simulink model "c10_wp_snake"  (R2021b)
settings: Solver=FixedStepDiscrete  StartTime=0.0  StopTime=Inf  FixedStep=sampleTime  RelTol=1e-3  EnableMultiTasking=on
InitFcn:
  | sampleTime = 0.05;
  | nMedianSize=3;
  | % Robot parameters
  | % Robot parameters
  | wheelRadius = 0.0303;
  | robotRadius = 0.116*0.8;   %小车在仿真中显示的圆形的半径大小
  | Trackwidth = 0.0847;  %定义向量场直方图算法中小车的宽度
  | 
  | % Lidar parameters
  | sensorOffset = [0,0];
  | scanAngles = linspace(-pi/3,pi/3,20)';%y = linspace(x1,x2,n) 生成 n 个点。这些点的间距为 (x2-x1)/(n-1)。
  | maxRange = 0.2;
  | 
  | %%%%%%
  | ks=1;
  | 
  | init_pose_1=[0    0  0]';
  | init_pose_2=[0    0.2  -pi/2]';
  | init_pose_3=[0    0.4  -pi/2]';
  | init_pose_4=[0    0.6  -pi/2]';
  | init_pose_5=[0    0.8  -pi/2]';
  | init_pose_6=[0    1  -pi/2]';
  | init_pose_7=[0    1.2  -pi/2]';
  | init_pose_8=[0    1.4  -pi/2]';
  | init_pose_9=[0    1.6  -pi/2]';
  | init_pose_10=[0   1.8  -pi/2]';
  | 
  | % paremeters of pure persuit
  | desired_v=0.2;
  | desired_w=2*pi;
  | desired_lookahead=0.2;
  | kv=0;
  | kw=1;%加速转弯
  | GoalRadius=0.15;%到达目标判定阈值
  | 
  | % paremeters of recovery
  | %recovery_w=0.5
  | recovery_w=2;
  | % Vector Field Histogram
  | numSector=180;%Number of angular sector
  | vehicleRadius=robotRadius;
  | rangeDis=[ 0, 0 ];%Range distance limits (m):
  | thresholds=[ 3, 8 ];%Histogram thresholds
  | %binary histogram 大于8是障碍物，小于3是空白区
  | %Thresholds for computing binary histogram, specified as a two-element vector of scalars. The algorithm uses these thresholds to compute the binary histogram from the polar obstacle density. Polar obstacle density values higher than the upper threshold are represented as occupied space (1) in the binary histogram. Values smaller than the lower threshold are represented as free space (0). Values that fall between the limits are set to the values of a previous computed binary histogram if one exists from previous iterations. If a previous histogram does not exist, the value is set as free space (0).
  | safetyDis=0.1;%Safety distance
  | minimumTurningRadius=0.5*robotRadius;%Minimum turning radius (m):
undefined symbols (not defined in the file): Angular, DiscIntNeverNeededParam, Linear
libraries: robotlib x42, dspstat3 x30, robotalgslib x20
(part 1 of 5)
settings Model: Creator=The MathWorks, Inc.  LastModifiedBy=FCS
settings SolverCC: AlgebraicLoopSolver=TrustRegion
settings DataIOCC: LimitDataPoints=on  SaveFormat=Array  ReturnWorkspaceOutputs=off
settings OptimizationCC: EnhancedBackFolding=on  PassReuseOutputArgsAs=Individual arguments  ZeroExternalMemoryAtStartup=off  ZeroInternalMemoryAtStartup=off  MaxStackSize=64  OptimizeBlockOrder=speed  DifferentSizesBufferReuse=on  OptimizationCustomize=off  EfficientTunableParamExpr=on
settings DebuggingCC: SolverPrmCheckMsg=warning  ParameterTunabilityLossMsg=error  SFUnexpectedBacktrackingDiag=warning  SFNoUnconditionalDefaultTransitionDiag=warning  SFExecutionAtInitializationDiag=none  SFMachineParentedDataDiag=warning  ArithmeticOperatorsInVariantConditions=warning
settings HardwareCC: ProdBitPerPointer=32  ProdBitPerSizeT=32  ProdBitPerPtrDiffT=32  ProdLargestAtomicFloat=None  ProdIntDivRoundTo=Undefined  ProdEndianess=Unspecified  ProdWordSize=32  ProdHWDeviceType=Generic->Unspecified (assume 32-bit Generic)  TargetHWDeviceType=Generic->Unspecified (assume 32-bit Generic)
settings ModelReferenceCC: PropagateSignalLabelsOutOfModel=off
settings SFSimCC: SimUseLocalCustomCode=off  MATLABDynamicMemAllocThreshold=655360  CustomCodeUndefinedFunction=UseInterfaceOnly  SimTargetLang=C++
settings RTWCC: Description=Embedded Coder  SystemTargetFile=ert.tlc  HardwareBoard=Robot Operating System (ROS)  TLCOptions="-aInlineSetEventsForThisBaseRateFcn=TLC_FALSE -aSuppressMultiTaskScheduler=TLC_FALSE  -aRateBasedStepFcn=0"  TemplateMakefile=ert_default_tmf  RTWUseLocalCustomCode=off  Toolchain=Catkin  TargetLang=C++
settings CodeAppCC: ForceParamTrailComments=on  IgnoreCustomStorageClasses=off  OperatorAnnotations=on  SimulinkDataObjDesc=on  SFDataObjDesc=on  InsertBlockDesc=on
settings ERTTargetCC: SupportVariableSizeSignals=on
settings ConfigComp: CovMetricSettings=dw  CovSaveCumulativeToWorkspaceVar=on  CovSaveSingleToWorkspaceVar=on  CovExternalEMLEnable=off  CovSFcnEnable=off

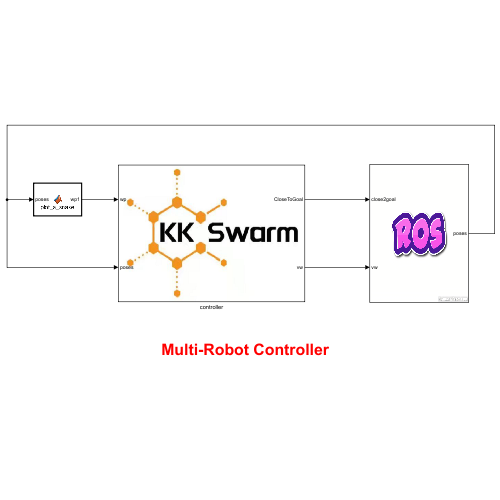
[thumbnail: Simulink's stored preview of the top-level diagram]
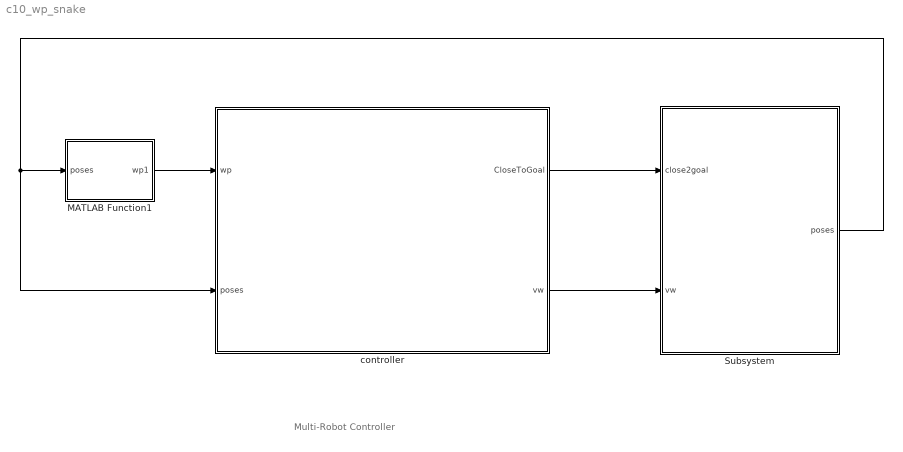
== system c10_wp_snake ==
  note: Multi-Robot Controller
  MATLAB Function1 : MATLAB Function  TreatAsAtomicUnit=on
  Subsystem : Subsystem
      mask Display: image('$imagefile'); % 使用工具条上的 "编辑图像" 进行更改。
  controller : Subsystem
      mask Display: image('$imagefile'); % 使用工具条上的 "编辑图像" 进行更改。
  wires:
  MATLAB Function1/1(wp1) -> controller/1(wp)
  controller/2(vw) -> Subsystem/2(vw)
  controller/1(CloseToGoal) -> Subsystem/1(close2goal)
  Subsystem/1(poses) -> controller/2(poses), MATLAB Function1/1(poses)

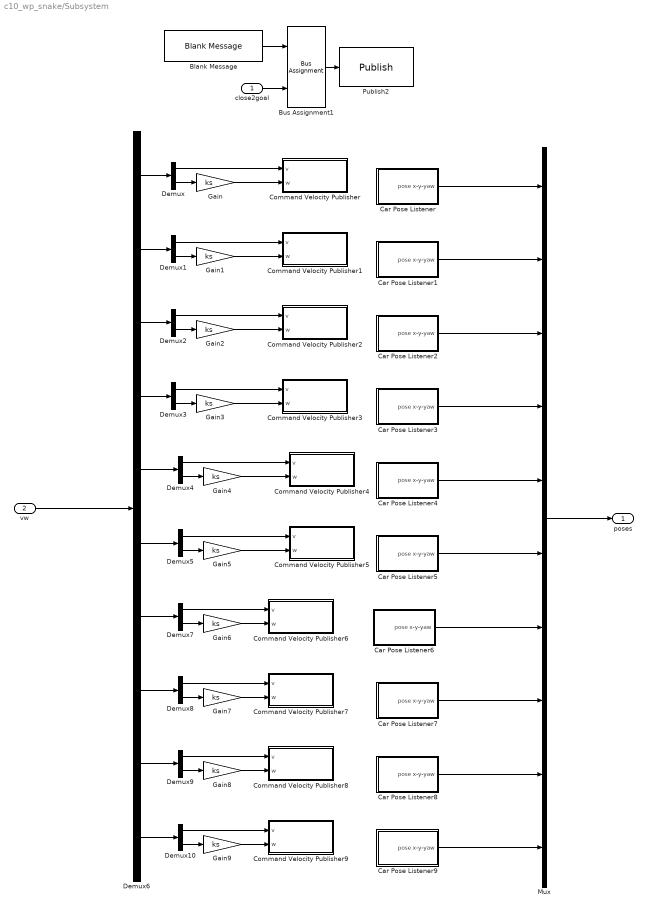
== system c10_wp_snake/Subsystem ==
  close2goal : Inport
  vw : Inport  Port=2
  Blank Message : robotlib/Blank Message  messageClass=Message  entityType=std_msgs/Float64  messageType=std_msgs/Float64  SampleTime=inf  legacyBusStruct=off
  Bus Assignment1 : BusAssignment  DialogController=Simulink.DDGSource_BusAssignment  AssignedSignals=Data
  Car Pose Listener : Subsystem
  Car Pose Listener1 : Subsystem
  Car Pose Listener2 : Subsystem
  Car Pose Listener3 : Subsystem
  Car Pose Listener4 : Subsystem
  Car Pose Listener5 : Subsystem
  Car Pose Listener6 : Subsystem
  Car Pose Listener7 : Subsystem
  Car Pose Listener8 : Subsystem
  Car Pose Listener9 : Subsystem
  Command Velocity Publisher : Subsystem
  Command Velocity Publisher1 : Subsystem
  Command Velocity Publisher2 : Subsystem
  Command Velocity Publisher3 : Subsystem
  Command Velocity Publisher4 : Subsystem
  Command Velocity Publisher5 : Subsystem
  Command Velocity Publisher6 : Subsystem
  Command Velocity Publisher7 : Subsystem
  Command Velocity Publisher8 : Subsystem
  Command Velocity Publisher9 : Subsystem
  Demux{,1..5,7..10} (10 alike) : Demux  Outputs=2
  Demux6 : Demux  Outputs=10
  Gain{,1..9} (10 alike) : Gain  Gain=ks
  Mux : Mux  Inputs=10
  Publish2 : robotlib/Publish  topicSource=Specify your own  topic=/close_goal  messageType=std_msgs/Float64  legacyBusStruct=off  messageQueueLength=105
  poses : Outport
  wires:
  Gain/1 -> Command Velocity Publisher/2(w)
  Demux/2 -> Gain/1
  Car Pose Listener/1(pose x-y-yaw) -> Mux/1
  Demux/1 -> Command Velocity Publisher/1(v)
  Car Pose Listener1/1(pose x-y-yaw) -> Mux/2
  Gain1/1 -> Command Velocity Publisher1/2(w)
  Demux1/2 -> Gain1/1
  Demux1/1 -> Command Velocity Publisher1/1(v)
  Car Pose Listener2/1(pose x-y-yaw) -> Mux/3
  Gain2/1 -> Command Velocity Publisher2/2(w)
  Demux2/2 -> Gain2/1
  Demux2/1 -> Command Velocity Publisher2/1(v)
  Car Pose Listener3/1(pose x-y-yaw) -> Mux/4
  Gain3/1 -> Command Velocity Publisher3/2(w)
  Demux3/2 -> Gain3/1
  Demux3/1 -> Command Velocity Publisher3/1(v)
  Gain4/1 -> Command Velocity Publisher4/2(w)
  Demux6/5 -> Demux4/1
  Demux4/2 -> Gain4/1
  Demux4/1 -> Command Velocity Publisher4/1(v)
  Car Pose Listener5/1(pose x-y-yaw) -> Mux/6
  Gain5/1 -> Command Velocity Publisher5/2(w)
  Demux6/6 -> Demux5/1
  Demux5/2 -> Gain5/1
  Demux5/1 -> Command Velocity Publisher5/1(v)
  Bus Assignment1/1 -> Publish2/1
  Blank Message/1 -> Bus Assignment1/1
  close2goal/1 -> Bus Assignment1/2
  Demux6/1 -> Demux/1
  Demux6/2 -> Demux1/1
  Demux6/3 -> Demux2/1
  Demux6/4 -> Demux3/1
  Car Pose Listener6/1(pose x-y-yaw) -> Mux/7
  Demux7/1 -> Command Velocity Publisher6/1(v)
  Demux7/2 -> Gain6/1
  Gain6/1 -> Command Velocity Publisher6/2(w)
  Demux6/7 -> Demux7/1
  Car Pose Listener7/1(pose x-y-yaw) -> Mux/8
  Demux8/1 -> Command Velocity Publisher7/1(v)
  Demux8/2 -> Gain7/1
  Gain7/1 -> Command Velocity Publisher7/2(w)
  Demux6/8 -> Demux8/1
  Car Pose Listener8/1(pose x-y-yaw) -> Mux/9
  Demux9/1 -> Command Velocity Publisher8/1(v)
  Demux9/2 -> Gain8/1
  Gain8/1 -> Command Velocity Publisher8/2(w)
  Demux6/9 -> Demux9/1
  Car Pose Listener9/1(pose x-y-yaw) -> Mux/10
  Demux10/1 -> Command Velocity Publisher9/1(v)
  Demux10/2 -> Gain9/1
  Gain9/1 -> Command Velocity Publisher9/2(w)
  Demux6/10 -> Demux10/1
  vw/1 -> Demux6/1
  Car Pose Listener4/1(pose x-y-yaw) -> Mux/5
  Mux/1 -> poses/1

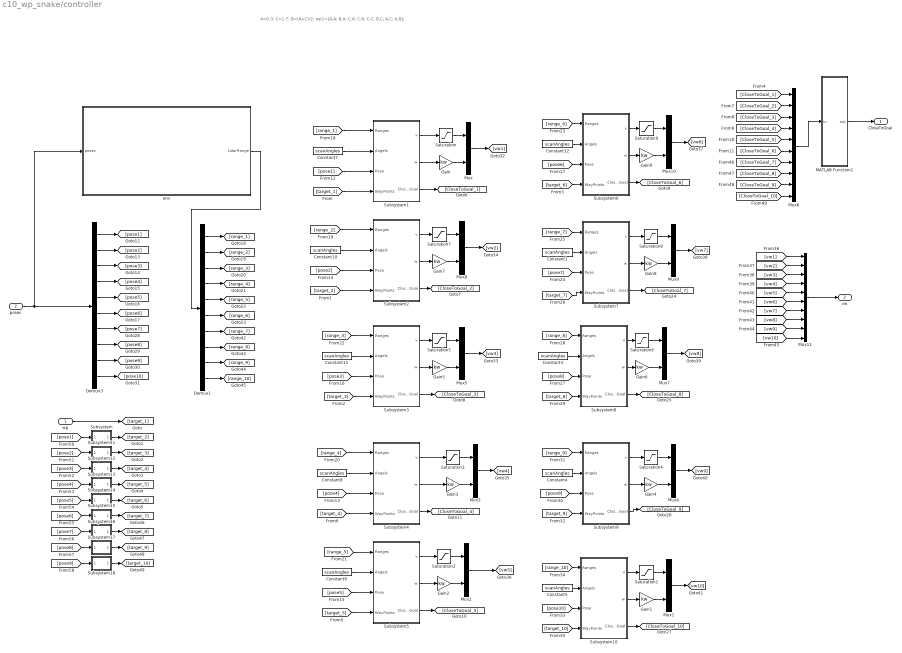
== system c10_wp_snake/controller ==
  note: A=0.3;
      | C=1.7;
      | B=(A+C)/2;
      |
      | wp1=[A,A; B,A; C,A;
      | C,B;
      | C,C; B,C; A,C;
      | A,B];
  wp : Inport
  poses : Inport  Port=2
  Constant{1,3..5,7..12} (10 alike) : Constant  Value=scanAngles
  Demux1 : Demux  Outputs=10
  Demux3 : Demux  Outputs=10
  Gain{,1..9} (10 alike) : Gain  Gain=kw
  MATLAB Function1 : MATLAB Function  TreatAsAtomicUnit=on
  Mux{,1..5,7..10} (10 alike) : Mux  Inputs=2
  Mux11 : Mux  Inputs=10
  Mux6 : Mux  Inputs=10
  Saturation{,1..9} (10 alike) : Saturate  UpperLimit=1  LowerLimit=0
  Subsystem : Subsystem
  Subsystem1 : Subsystem
  Subsystem10 : Subsystem
  Subsystem11 : Subsystem
  Subsystem12 : Subsystem
  Subsystem13 : Subsystem
  Subsystem14 : Subsystem
  Subsystem15 : Subsystem
  Subsystem16 : Subsystem
  Subsystem17 : Subsystem
  Subsystem18 : Subsystem
  Subsystem2 : Subsystem
  Subsystem3 : Subsystem
  Subsystem4 : Subsystem
  Subsystem5 : Subsystem
  Subsystem6 : Subsystem
  Subsystem7 : Subsystem
  Subsystem8 : Subsystem
  Subsystem9 : Subsystem
  env : Subsystem
      mask Display: image('$imagefile'); % 使用工具条上的 "编辑图像" 进行更改。
  CloseToGoal : Outport
  vw : Outport  Port=2
  wires:
  [pose3] -> Subsystem12/1(In1)
  [range_3] -> Subsystem3/1(Ranges)
  Subsystem4/3(CloseToGoal) -> [CloseToGoal_4]
  [pose1] -> Subsystem/1(In1)
  Saturation/1 -> Mux/1
  Subsystem1/3(CloseToGoal) -> [CloseToGoal_1]
  Subsystem3/3(CloseToGoal) -> [CloseToGoal_3]
  Subsystem5/3(CloseToGoal) -> [CloseToGoal_5]
  Subsystem6/3(CloseToGoal) -> [CloseToGoal_6]
  [target_3] -> Subsystem3/4(WayPoints)
  Subsystem2/3(CloseToGoal) -> [CloseToGoal_2]
  Constant10/1 -> Subsystem2/2(Angels)
  [pose2] -> Subsystem2/3(Pose)
  Constant7/1 -> Subsystem1/2(Angels)
  Constant11/1 -> Subsystem3/2(Angels)
  [range_6] -> Subsystem6/1(Ranges)
  wp/1 -> [target_1]
  [pose2] -> Subsystem11/1(In1)
  [pose4] -> Subsystem13/1(In1)
  Constant9/1 -> Subsystem5/2(Angels)
  [target_6] -> Subsystem6/4(WayPoints)
  [pose5] -> Subsystem14/1(In1)
  Gain/1 -> Mux/2
  [pose5] -> Subsystem5/3(Pose)
  [pose3] -> Subsystem3/3(Pose)
  [target_4] -> Subsystem4/4(WayPoints)
  [range_4] -> Subsystem4/1(Ranges)
  Constant8/1 -> Subsystem4/2(Angels)
  Constant12/1 -> Subsystem6/2(Angels)
  [target_2] -> Subsystem2/4(WayPoints)
  [target_1] -> Subsystem1/4(WayPoints)
  Subsystem1/1(v) -> Saturation/1
  [target_5] -> Subsystem5/4(WayPoints)
  [range_5] -> Subsystem5/1(Ranges)
  [pose6] -> Subsystem6/3(Pose)
  [pose1] -> Subsystem1/3(Pose)
  Mux/1 -> [vw1]
  [pose4] -> Subsystem4/3(Pose)
  [CloseToGoal_2] -> Mux6/2
  [CloseToGoal_6] -> Mux6/6
  [CloseToGoal_3] -> Mux6/3
  [CloseToGoal_1] -> Mux6/1
  MATLAB Function1/1(out) -> CloseToGoal/1
  Mux6/1 -> MATLAB Function1/1(in)
  [CloseToGoal_4] -> Mux6/4
  [CloseToGoal_5] -> Mux6/5
  Demux3/3 -> [pose3]
  Demux3/6 -> [pose6]
  Demux3/1 -> [pose1]
  Demux3/5 -> [pose5]
  Demux3/2 -> [pose2]
  Demux3/4 -> [pose4]
  poses/1 -> Demux3/1, env/1(poses)
  Demux1/3 -> [range_3]
  Demux1/2 -> [range_2]
  Demux1/1 -> [range_1]
  Demux1/4 -> [range_4]
  Demux1/6 -> [range_6]
  Demux1/5 -> [range_5]
  env/1(LidarRange) -> Demux1/1
  [range_1] -> Subsystem1/1(Ranges)
  [range_2] -> Subsystem2/1(Ranges)
  [range_7] -> Subsystem7/1(Ranges)
  Constant1/1 -> Subsystem7/2(Angels)
  [target_7] -> Subsystem7/4(WayPoints)
  Subsystem7/3(CloseToGoal) -> [CloseToGoal_7]
  [pose7] -> Subsystem7/3(Pose)
  [range_8] -> Subsystem8/1(Ranges)
  Constant3/1 -> Subsystem8/2(Angels)
  [target_8] -> Subsystem8/4(WayPoints)
  Subsystem8/3(CloseToGoal) -> [CloseToGoal_8]
  [pose8] -> Subsystem8/3(Pose)
  [range_9] -> Subsystem9/1(Ranges)
  Constant4/1 -> Subsystem9/2(Angels)
  [target_9] -> Subsystem9/4(WayPoints)
  Subsystem9/3(CloseToGoal) -> [CloseToGoal_9]
  [range_10] -> Subsystem10/1(Ranges)
  Constant5/1 -> Subsystem10/2(Angels)
  [target_10] -> Subsystem10/4(WayPoints)
  Subsystem10/3(CloseToGoal) -> [CloseToGoal_10]
  [pose10] -> Subsystem10/3(Pose)
  Demux3/7 -> [pose7]
  Demux3/8 -> [pose8]
  Demux3/9 -> [pose9]
  Demux3/10 -> [pose10]
  [vw1] -> Mux11/1
  [vw2] -> Mux11/2
  [vw3] -> Mux11/3
  [vw4] -> Mux11/4
  [vw5] -> Mux11/5
  [vw6] -> Mux11/6
  [vw7] -> Mux11/7
  [vw8] -> Mux11/8
  [vw9] -> Mux11/9
  [vw10] -> Mux11/10
  Mux11/1 -> vw/1
  Demux1/7 -> [range_7]
  Demux1/8 -> [range_8]
  Demux1/9 -> [range_9]
  Demux1/10 -> [range_10]
  [pose6] -> Subsystem15/1(In1)
  [pose7] -> Subsystem16/1(In1)
  [pose8] -> Subsystem17/1(In1)
  [pose9] -> Subsystem18/1(In1)
  [pose9] -> Subsystem9/3(Pose)
  Subsystem1/2(w) -> Gain/1
  [CloseToGoal_7] -> Mux6/7
  [CloseToGoal_9] -> Mux6/9
  [CloseToGoal_10] -> Mux6/10
  [CloseToGoal_8] -> Mux6/8
  Gain1/1 -> Mux1/2
  Mux1/1 -> [vw10]
  Saturation1/1 -> Mux1/1
  Subsystem10/1(v) -> Saturation1/1
  Subsystem10/2(w) -> Gain1/1
  Gain2/1 -> Mux2/2
  Mux2/1 -> [vw5]
  Saturation2/1 -> Mux2/1
  Subsystem5/1(v) -> Saturation2/1
  Subsystem5/2(w) -> Gain2/1
  Gain3/1 -> Mux3/2
  Mux3/1 -> [vw4]
  Saturation3/1 -> Mux3/1
  Subsystem4/1(v) -> Saturation3/1
  Subsystem4/2(w) -> Gain3/1
  Gain4/1 -> Mux4/2
  Mux4/1 -> [vw9]
  Saturation4/1 -> Mux4/1
  Subsystem9/1(v) -> Saturation4/1
  Subsystem9/2(w) -> Gain4/1
  Gain5/1 -> Mux5/2
  Mux5/1 -> [vw3]
  Saturation5/1 -> Mux5/1
  Subsystem3/1(v) -> Saturation5/1
  Subsystem3/2(w) -> Gain5/1
  Gain6/1 -> Mux7/2
  Mux7/1 -> [vw8]
  Saturation6/1 -> Mux7/1
  Subsystem8/1(v) -> Saturation6/1
  Subsystem8/2(w) -> Gain6/1
  Gain7/1 -> Mux8/2
  Mux8/1 -> [vw2]
  Saturation7/1 -> Mux8/1
  Subsystem2/1(v) -> Saturation7/1
  Subsystem2/2(w) -> Gain7/1
  Gain8/1 -> Mux9/2
  Mux9/1 -> [vw7]
  Saturation8/1 -> Mux9/1
  Subsystem7/1(v) -> Saturation8/1
  Subsystem7/2(w) -> Gain8/1
  Gain9/1 -> Mux10/2
  Mux10/1 -> [vw6]
  Saturation9/1 -> Mux10/1
  Subsystem6/1(v) -> Saturation9/1
  Subsystem6/2(w) -> Gain9/1
  Subsystem/1(Out1) -> [target_2]
  Subsystem11/1(Out1) -> [target_3]
  Subsystem12/1(Out1) -> [target_4]
  Subsystem13/1(Out1) -> [target_5]
  Subsystem14/1(Out1) -> [target_6]
  Subsystem15/1(Out1) -> [target_7]
  Subsystem16/1(Out1) -> [target_8]
  Subsystem17/1(Out1) -> [target_9]
  Subsystem18/1(Out1) -> [target_10]

== system c10_wp_snake/Subsystem/Car Pose Listener ==
  Subscribe : robotlib/Subscribe  topicSource=Specify your own  topic=/robot_1/pose  messageType=nav_msgs/Odometry  SampleTime=-1  legacyBusStruct=off  messageQueueLength=51
  Subscribe1 : robotlib/Subscribe  topicSource=Specify your own  topic=/robot_1/odometry  messageType=geometry_msgs/Twist  SampleTime=-1  legacyBusStruct=off  messageQueueLength=51
  Subsystem : Subsystem
  pose x-y-yaw : Outport
  wires:
  Subscribe/1 -> Subsystem/1(poseNew)  "IsNew"
  Subscribe/2 -> Subsystem/2(poseMsg)
  Subscribe1/1 -> Subsystem/3(VW_New)  "IsNew"
  Subscribe1/2 -> Subsystem/4(VW_Msg)
  Subsystem/1(pose) -> pose x-y-yaw/1

== system c10_wp_snake/Subsystem/Car Pose Listener1 ==
  Subscribe : robotlib/Subscribe  topicSource=Specify your own  topic=/robot_2/pose  messageType=nav_msgs/Odometry  SampleTime=-1  legacyBusStruct=off  messageQueueLength=51
  Subscribe1 : robotlib/Subscribe  topicSource=Specify your own  topic=/robot_2/odometry  messageType=geometry_msgs/Twist  SampleTime=-1  legacyBusStruct=off  messageQueueLength=51
  Subsystem : Subsystem
  pose x-y-yaw : Outport
  wires:
  Subscribe/1 -> Subsystem/1(poseNew)  "IsNew"
  Subscribe/2 -> Subsystem/2(poseMsg)
  Subscribe1/2 -> Subsystem/4(VW_Msg)
  Subscribe1/1 -> Subsystem/3(VW_New)  "IsNew"
  Subsystem/1(pose) -> pose x-y-yaw/1

== system c10_wp_snake/Subsystem/Car Pose Listener2 ==
  Subscribe : robotlib/Subscribe  topicSource=Specify your own  topic=/robot_3/pose  messageType=nav_msgs/Odometry  SampleTime=-1  legacyBusStruct=off  messageQueueLength=51
  Subscribe1 : robotlib/Subscribe  topicSource=Specify your own  topic=/robot_3/odometry  messageType=geometry_msgs/Twist  SampleTime=-1  legacyBusStruct=off  messageQueueLength=51
  Subsystem : Subsystem
  pose x-y-yaw : Outport
  wires:
  Subscribe/1 -> Subsystem/1(poseNew)  "IsNew"
  Subscribe/2 -> Subsystem/2(poseMsg)
  Subscribe1/1 -> Subsystem/3(VW_New)  "IsNew"
  Subscribe1/2 -> Subsystem/4(VW_Msg)
  Subsystem/1(pose) -> pose x-y-yaw/1

== system c10_wp_snake/Subsystem/Car Pose Listener3 ==
  Subscribe : robotlib/Subscribe  topicSource=Specify your own  topic=/robot_4/pose  messageType=nav_msgs/Odometry  SampleTime=-1  legacyBusStruct=off  messageQueueLength=51
  Subscribe1 : robotlib/Subscribe  topicSource=Specify your own  topic=/robot_4/odometry  messageType=geometry_msgs/Twist  SampleTime=-1  legacyBusStruct=off  messageQueueLength=51
  Subsystem : Subsystem
  pose x-y-yaw : Outport
  wires:
  Subscribe/1 -> Subsystem/1(poseNew)  "IsNew"
  Subscribe/2 -> Subsystem/2(poseMsg)
  Subscribe1/1 -> Subsystem/3(VW_New)  "IsNew"
  Subscribe1/2 -> Subsystem/4(VW_Msg)
  Subsystem/1(pose) -> pose x-y-yaw/1

== system c10_wp_snake/Subsystem/Car Pose Listener4 ==
  Subscribe : robotlib/Subscribe  topicSource=Specify your own  topic=/robot_5/pose  messageType=nav_msgs/Odometry  SampleTime=-1  legacyBusStruct=off  messageQueueLength=51
  Subscribe1 : robotlib/Subscribe  topicSource=Specify your own  topic=/robot_5/odometry  messageType=geometry_msgs/Twist  SampleTime=-1  legacyBusStruct=off  messageQueueLength=51
  Subsystem : Subsystem
  pose x-y-yaw : Outport
  wires:
  Subscribe/1 -> Subsystem/1(poseNew)  "IsNew"
  Subscribe/2 -> Subsystem/2(poseMsg)
  Subscribe1/1 -> Subsystem/3(VW_New)  "IsNew"
  Subscribe1/2 -> Subsystem/4(VW_Msg)
  Subsystem/1(pose) -> pose x-y-yaw/1

== system c10_wp_snake/Subsystem/Car Pose Listener5 ==
  Subscribe : robotlib/Subscribe  topicSource=Specify your own  topic=/robot_6/pose  messageType=nav_msgs/Odometry  SampleTime=-1  legacyBusStruct=off  messageQueueLength=51
  Subscribe1 : robotlib/Subscribe  topicSource=Specify your own  topic=/robot_6/odometry  messageType=geometry_msgs/Twist  SampleTime=-1  legacyBusStruct=off  messageQueueLength=51
  Subsystem : Subsystem
  pose x-y-yaw : Outport
  wires:
  Subscribe/1 -> Subsystem/1(poseNew)  "IsNew"
  Subscribe/2 -> Subsystem/2(poseMsg)
  Subscribe1/1 -> Subsystem/3(VW_New)  "IsNew"
  Subscribe1/2 -> Subsystem/4(VW_Msg)
  Subsystem/1(pose) -> pose x-y-yaw/1

== system c10_wp_snake/Subsystem/Car Pose Listener6 ==
  Subscribe : robotlib/Subscribe  topicSource=Specify your own  topic=/robot_7/pose  messageType=nav_msgs/Odometry  SampleTime=-1  legacyBusStruct=off  messageQueueLength=51
  Subscribe1 : robotlib/Subscribe  topicSource=Specify your own  topic=/robot_7/odometry  messageType=geometry_msgs/Twist  SampleTime=-1  legacyBusStruct=off  messageQueueLength=51
  Subsystem : Subsystem
  pose x-y-yaw : Outport
  wires:
  Subsystem/1(pose) -> pose x-y-yaw/1
  Subscribe1/2 -> Subsystem/4(VW_Msg)
  Subscribe1/1 -> Subsystem/3(VW_New)  "IsNew"
  Subscribe/2 -> Subsystem/2(poseMsg)
  Subscribe/1 -> Subsystem/1(poseNew)  "IsNew"

== system c10_wp_snake/Subsystem/Car Pose Listener7 ==
  Subscribe : robotlib/Subscribe  topicSource=Specify your own  topic=/robot_8/pose  messageType=nav_msgs/Odometry  SampleTime=-1  legacyBusStruct=off  messageQueueLength=51
  Subscribe1 : robotlib/Subscribe  topicSource=Specify your own  topic=/robot_8/odometry  messageType=geometry_msgs/Twist  SampleTime=-1  legacyBusStruct=off  messageQueueLength=51
  Subsystem : Subsystem
  pose x-y-yaw : Outport
  wires:
  Subscribe/1 -> Subsystem/1(poseNew)  "IsNew"
  Subscribe/2 -> Subsystem/2(poseMsg)
  Subscribe1/1 -> Subsystem/3(VW_New)  "IsNew"
  Subscribe1/2 -> Subsystem/4(VW_Msg)
  Subsystem/1(pose) -> pose x-y-yaw/1

== system c10_wp_snake/Subsystem/Car Pose Listener8 ==
  Subscribe : robotlib/Subscribe  topicSource=Specify your own  topic=/robot_9/pose  messageType=nav_msgs/Odometry  SampleTime=-1  legacyBusStruct=off  messageQueueLength=51
  Subscribe1 : robotlib/Subscribe  topicSource=Specify your own  topic=/robot_9/odometry  messageType=geometry_msgs/Twist  SampleTime=-1  legacyBusStruct=off  messageQueueLength=51
  Subsystem : Subsystem
  pose x-y-yaw : Outport
  wires:
  Subsystem/1(pose) -> pose x-y-yaw/1
  Subscribe1/2 -> Subsystem/4(VW_Msg)
  Subscribe1/1 -> Subsystem/3(VW_New)  "IsNew"
  Subscribe/2 -> Subsystem/2(poseMsg)
  Subscribe/1 -> Subsystem/1(poseNew)  "IsNew"

== system c10_wp_snake/Subsystem/Car Pose Listener9 ==
  Subscribe : robotlib/Subscribe  topicSource=Specify your own  topic=/robot_10/pose  messageType=nav_msgs/Odometry  SampleTime=-1  legacyBusStruct=off  messageQueueLength=51
  Subscribe1 : robotlib/Subscribe  topicSource=Specify your own  topic=/robot_10/odometry  messageType=geometry_msgs/Twist  SampleTime=-1  legacyBusStruct=off  messageQueueLength=51
  Subsystem : Subsystem
  pose x-y-yaw : Outport
  wires:
  Subscribe/1 -> Subsystem/1(poseNew)  "IsNew"
  Subscribe/2 -> Subsystem/2(poseMsg)
  Subscribe1/1 -> Subsystem/3(VW_New)  "IsNew"
  Subscribe1/2 -> Subsystem/4(VW_Msg)
  Subsystem/1(pose) -> pose x-y-yaw/1

== system c10_wp_snake/Subsystem/Command Velocity Publisher ==
  v : Inport
  w : Inport  Port=2
  Blank Message : robotlib/Blank Message  messageClass=Message  entityType=geometry_msgs/Twist  messageType=geometry_msgs/Twist  SampleTime=inf  legacyBusStruct=off
  Bus Assignment1 : BusAssignment  DialogController=Simulink.DDGSource_BusAssignment  AssignedSignals=Linear.X,Angular.Z
  Publish2 : robotlib/Publish  topicSource=Specify your own  topic=/robot_1/cmd_vel  messageType=geometry_msgs/Twist  legacyBusStruct=off  messageQueueLength=105
  wires:
  Bus Assignment1/1 -> Publish2/1
  Blank Message/1 -> Bus Assignment1/1
  v/1 -> Bus Assignment1/2
  w/1 -> Bus Assignment1/3

== system c10_wp_snake/Subsystem/Command Velocity Publisher1 ==
  v : Inport
  w : Inport  Port=2
  Blank Message : robotlib/Blank Message  messageClass=Message  entityType=geometry_msgs/Twist  messageType=geometry_msgs/Twist  SampleTime=inf  legacyBusStruct=off
  Bus Assignment1 : BusAssignment  DialogController=Simulink.DDGSource_BusAssignment  AssignedSignals=Linear.X,Angular.Z
  Publish2 : robotlib/Publish  topicSource=Specify your own  topic=/robot_2/cmd_vel  messageType=geometry_msgs/Twist  legacyBusStruct=off  messageQueueLength=105
  wires:
  Bus Assignment1/1 -> Publish2/1
  Blank Message/1 -> Bus Assignment1/1
  v/1 -> Bus Assignment1/2
  w/1 -> Bus Assignment1/3

== system c10_wp_snake/Subsystem/Command Velocity Publisher2 ==
  v : Inport
  w : Inport  Port=2
  Blank Message : robotlib/Blank Message  messageClass=Message  entityType=geometry_msgs/Twist  messageType=geometry_msgs/Twist  SampleTime=inf  legacyBusStruct=off
  Bus Assignment1 : BusAssignment  DialogController=Simulink.DDGSource_BusAssignment  AssignedSignals=Linear.X,Angular.Z
  Publish2 : robotlib/Publish  topicSource=Specify your own  topic=/robot_3/cmd_vel  messageType=geometry_msgs/Twist  legacyBusStruct=off  messageQueueLength=105
  wires:
  Bus Assignment1/1 -> Publish2/1
  Blank Message/1 -> Bus Assignment1/1
  v/1 -> Bus Assignment1/2
  w/1 -> Bus Assignment1/3

== system c10_wp_snake/Subsystem/Command Velocity Publisher3 ==
  v : Inport
  w : Inport  Port=2
  Blank Message : robotlib/Blank Message  messageClass=Message  entityType=geometry_msgs/Twist  messageType=geometry_msgs/Twist  SampleTime=inf  legacyBusStruct=off
  Bus Assignment1 : BusAssignment  DialogController=Simulink.DDGSource_BusAssignment  AssignedSignals=Linear.X,Angular.Z
  Publish2 : robotlib/Publish  topicSource=Specify your own  topic=/robot_4/cmd_vel  messageType=geometry_msgs/Twist  legacyBusStruct=off  messageQueueLength=105
  wires:
  Bus Assignment1/1 -> Publish2/1
  Blank Message/1 -> Bus Assignment1/1
  v/1 -> Bus Assignment1/2
  w/1 -> Bus Assignment1/3

== system c10_wp_snake/Subsystem/Command Velocity Publisher4 ==
  v : Inport
  w : Inport  Port=2
  Blank Message : robotlib/Blank Message  messageClass=Message  entityType=geometry_msgs/Twist  messageType=geometry_msgs/Twist  SampleTime=inf  legacyBusStruct=off
  Bus Assignment1 : BusAssignment  DialogController=Simulink.DDGSource_BusAssignment  AssignedSignals=Linear.X,Angular.Z
  Publish2 : robotlib/Publish  topicSource=Specify your own  topic=/robot_5/cmd_vel  messageType=geometry_msgs/Twist  legacyBusStruct=off  messageQueueLength=105
  wires:
  Bus Assignment1/1 -> Publish2/1
  Blank Message/1 -> Bus Assignment1/1
  v/1 -> Bus Assignment1/2
  w/1 -> Bus Assignment1/3

== system c10_wp_snake/Subsystem/Command Velocity Publisher5 ==
  v : Inport
  w : Inport  Port=2
  Blank Message : robotlib/Blank Message  messageClass=Message  entityType=geometry_msgs/Twist  messageType=geometry_msgs/Twist  SampleTime=inf  legacyBusStruct=off
  Bus Assignment1 : BusAssignment  DialogController=Simulink.DDGSource_BusAssignment  AssignedSignals=Linear.X,Angular.Z
  Publish2 : robotlib/Publish  topicSource=Specify your own  topic=/robot_6/cmd_vel  messageType=geometry_msgs/Twist  legacyBusStruct=off  messageQueueLength=105
  wires:
  Bus Assignment1/1 -> Publish2/1
  Blank Message/1 -> Bus Assignment1/1
  v/1 -> Bus Assignment1/2
  w/1 -> Bus Assignment1/3

== system c10_wp_snake/Subsystem/Command Velocity Publisher6 ==
  v : Inport
  w : Inport  Port=2
  Blank Message : robotlib/Blank Message  messageClass=Message  entityType=geometry_msgs/Twist  messageType=geometry_msgs/Twist  SampleTime=inf  legacyBusStruct=off
  Bus Assignment1 : BusAssignment  DialogController=Simulink.DDGSource_BusAssignment  AssignedSignals=Linear.X,Angular.Z
  Publish2 : robotlib/Publish  topicSource=Specify your own  topic=/robot_7/cmd_vel  messageType=geometry_msgs/Twist  legacyBusStruct=off  messageQueueLength=105
  wires:
  w/1 -> Bus Assignment1/3
  v/1 -> Bus Assignment1/2
  Blank Message/1 -> Bus Assignment1/1
  Bus Assignment1/1 -> Publish2/1

== system c10_wp_snake/Subsystem/Command Velocity Publisher7 ==
  v : Inport
  w : Inport  Port=2
  Blank Message : robotlib/Blank Message  messageClass=Message  entityType=geometry_msgs/Twist  messageType=geometry_msgs/Twist  SampleTime=inf  legacyBusStruct=off
  Bus Assignment1 : BusAssignment  DialogController=Simulink.DDGSource_BusAssignment  AssignedSignals=Linear.X,Angular.Z
  Publish2 : robotlib/Publish  topicSource=Specify your own  topic=/robot_8/cmd_vel  messageType=geometry_msgs/Twist  legacyBusStruct=off  messageQueueLength=105
  wires:
  Bus Assignment1/1 -> Publish2/1
  Blank Message/1 -> Bus Assignment1/1
  v/1 -> Bus Assignment1/2
  w/1 -> Bus Assignment1/3

== system c10_wp_snake/Subsystem/Command Velocity Publisher8 ==
  v : Inport
  w : Inport  Port=2
  Blank Message : robotlib/Blank Message  messageClass=Message  entityType=geometry_msgs/Twist  messageType=geometry_msgs/Twist  SampleTime=inf  legacyBusStruct=off
  Bus Assignment1 : BusAssignment  DialogController=Simulink.DDGSource_BusAssignment  AssignedSignals=Linear.X,Angular.Z
  Publish2 : robotlib/Publish  topicSource=Specify your own  topic=/robot_9/cmd_vel  messageType=geometry_msgs/Twist  legacyBusStruct=off  messageQueueLength=105
  wires:
  w/1 -> Bus Assignment1/3
  v/1 -> Bus Assignment1/2
  Blank Message/1 -> Bus Assignment1/1
  Bus Assignment1/1 -> Publish2/1

== system c10_wp_snake/Subsystem/Command Velocity Publisher9 ==
  v : Inport
  w : Inport  Port=2
  Blank Message : robotlib/Blank Message  messageClass=Message  entityType=geometry_msgs/Twist  messageType=geometry_msgs/Twist  SampleTime=inf  legacyBusStruct=off
  Bus Assignment1 : BusAssignment  DialogController=Simulink.DDGSource_BusAssignment  AssignedSignals=Linear.X,Angular.Z
  Publish2 : robotlib/Publish  topicSource=Specify your own  topic=/robot_10/cmd_vel  messageType=geometry_msgs/Twist  legacyBusStruct=off  messageQueueLength=105
  wires:
  Bus Assignment1/1 -> Publish2/1
  Blank Message/1 -> Bus Assignment1/1
  v/1 -> Bus Assignment1/2
  w/1 -> Bus Assignment1/3

== system c10_wp_snake/controller/Subsystem ==
  In1 : Inport
  Demux1 : Demux  Outputs=3
  Mux5 : Mux  Inputs=2
  Reshape : Reshape  OutputDimensionality=Customize  OutputDimensions=[1,2]
  Terminator : Terminator
  Out1 : Outport
  wires:
  In1/1 -> Demux1/1
  Demux1/1 -> Mux5/1
  Demux1/2 -> Mux5/2
  Demux1/3 -> Terminator/1
  Mux5/1 -> Reshape/1
  Reshape/1 -> Out1/1

== system c10_wp_snake/controller/Subsystem1 ==
  note: Path Following with Obstacle Avoidance in Simulink
  Ranges : Inport
  Angels : Inport  Port=2
  Pose : Inport  Port=3
  WayPoints : Inport  Port=4
  Adjust Velocities to Avoid Obstacles : Subsystem
  Compute Velocity and Heading for Path following : Subsystem
  Constant1 : Constant  Value=scanAngles
  More Info : Subsystem
      settings: OpenFcn=showdemo(bdroot(gcb))
      mask Display: disp('?')
  Outputs : Subsystem
  v : Outport
  w : Outport  Port=2
  CloseToGoal : Outport  Port=3
  wires:
  Angels/1 -> Adjust Velocities to Avoid Obstacles/2(Angles)
  Compute Velocity and Heading for Path following/1(TargetDir) -> Adjust Velocities to Avoid Obstacles/3(TargetDir)
  Compute Velocity and Heading for Path following/3(W) -> Outputs/4(W), Adjust Velocities to Avoid Obstacles/5(W)
  Pose/1 -> Compute Velocity and Heading for Path following/1(CurrentPose)
  Adjust Velocities to Avoid Obstacles/2(dW) -> Outputs/2(dW)
  Compute Velocity and Heading for Path following/2(V) -> Outputs/3(V), Adjust Velocities to Avoid Obstacles/4(V)
  Ranges/1 -> Adjust Velocities to Avoid Obstacles/1(Ranges)
  WayPoints/1 -> Compute Velocity and Heading for Path following/2(Waypoints)
  Compute Velocity and Heading for Path following/4(CloseToGoal) -> Outputs/5(CloseToGoal), CloseToGoal/1
  Adjust Velocities to Avoid Obstacles/1(dV) -> Outputs/1(dV)
  Outputs/1(v) -> v/1
  Outputs/2(w) -> w/1

== system c10_wp_snake/controller/Subsystem10 ==
  note: Path Following with Obstacle Avoidance in Simulink
  Ranges : Inport
  Angels : Inport  Port=2
  Pose : Inport  Port=3
  WayPoints : Inport  Port=4
  Adjust Velocities to Avoid Obstacles : Subsystem
  Compute Velocity and Heading for Path following : Subsystem
  Constant1 : Constant  Value=scanAngles
  More Info : Subsystem
      settings: OpenFcn=showdemo(bdroot(gcb))
      mask Display: disp('?')
  Outputs : Subsystem
  v : Outport
  w : Outport  Port=2
  CloseToGoal : Outport  Port=3
  wires:
  Outputs/2(w) -> w/1
  Outputs/1(v) -> v/1
  Adjust Velocities to Avoid Obstacles/1(dV) -> Outputs/1(dV)
  Compute Velocity and Heading for Path following/4(CloseToGoal) -> CloseToGoal/1, Outputs/5(CloseToGoal)
  WayPoints/1 -> Compute Velocity and Heading for Path following/2(Waypoints)
  Ranges/1 -> Adjust Velocities to Avoid Obstacles/1(Ranges)
  Compute Velocity and Heading for Path following/2(V) -> Adjust Velocities to Avoid Obstacles/4(V), Outputs/3(V)
  Adjust Velocities to Avoid Obstacles/2(dW) -> Outputs/2(dW)
  Pose/1 -> Compute Velocity and Heading for Path following/1(CurrentPose)
  Compute Velocity and Heading for Path following/3(W) -> Adjust Velocities to Avoid Obstacles/5(W), Outputs/4(W)
  Compute Velocity and Heading for Path following/1(TargetDir) -> Adjust Velocities to Avoid Obstacles/3(TargetDir)
  Angels/1 -> Adjust Velocities to Avoid Obstacles/2(Angles)

== system c10_wp_snake/controller/Subsystem11 ==
  In1 : Inport
  Demux1 : Demux  Outputs=3
  Mux5 : Mux  Inputs=2
  Reshape : Reshape  OutputDimensionality=Customize  OutputDimensions=[1,2]
  Terminator : Terminator
  Out1 : Outport
  wires:
  Reshape/1 -> Out1/1
  Mux5/1 -> Reshape/1
  Demux1/3 -> Terminator/1
  Demux1/2 -> Mux5/2
  Demux1/1 -> Mux5/1
  In1/1 -> Demux1/1

== system c10_wp_snake/controller/Subsystem12 ==
  In1 : Inport
  Demux1 : Demux  Outputs=3
  Mux5 : Mux  Inputs=2
  Reshape : Reshape  OutputDimensionality=Customize  OutputDimensions=[1,2]
  Terminator : Terminator
  Out1 : Outport
  wires:
  In1/1 -> Demux1/1
  Demux1/1 -> Mux5/1
  Demux1/2 -> Mux5/2
  Demux1/3 -> Terminator/1
  Mux5/1 -> Reshape/1
  Reshape/1 -> Out1/1

== system c10_wp_snake/controller/Subsystem13 ==
  In1 : Inport
  Demux1 : Demux  Outputs=3
  Mux5 : Mux  Inputs=2
  Reshape : Reshape  OutputDimensionality=Customize  OutputDimensions=[1,2]
  Terminator : Terminator
  Out1 : Outport
  wires:
  Reshape/1 -> Out1/1
  Mux5/1 -> Reshape/1
  Demux1/3 -> Terminator/1
  Demux1/2 -> Mux5/2
  Demux1/1 -> Mux5/1
  In1/1 -> Demux1/1

== system c10_wp_snake/controller/Subsystem14 ==
  In1 : Inport
  Demux1 : Demux  Outputs=3
  Mux5 : Mux  Inputs=2
  Reshape : Reshape  OutputDimensionality=Customize  OutputDimensions=[1,2]
  Terminator : Terminator
  Out1 : Outport
  wires:
  In1/1 -> Demux1/1
  Demux1/1 -> Mux5/1
  Demux1/2 -> Mux5/2
  Demux1/3 -> Terminator/1
  Mux5/1 -> Reshape/1
  Reshape/1 -> Out1/1

== system c10_wp_snake/controller/Subsystem15 ==
  In1 : Inport
  Demux1 : Demux  Outputs=3
  Mux5 : Mux  Inputs=2
  Reshape : Reshape  OutputDimensionality=Customize  OutputDimensions=[1,2]
  Terminator : Terminator
  Out1 : Outport
  wires:
  Reshape/1 -> Out1/1
  Mux5/1 -> Reshape/1
  Demux1/3 -> Terminator/1
  Demux1/2 -> Mux5/2
  Demux1/1 -> Mux5/1
  In1/1 -> Demux1/1

== system c10_wp_snake/controller/Subsystem16 ==
  In1 : Inport
  Demux1 : Demux  Outputs=3
  Mux5 : Mux  Inputs=2
  Reshape : Reshape  OutputDimensionality=Customize  OutputDimensions=[1,2]
  Terminator : Terminator
  Out1 : Outport
  wires:
  In1/1 -> Demux1/1
  Demux1/1 -> Mux5/1
  Demux1/2 -> Mux5/2
  Demux1/3 -> Terminator/1
  Mux5/1 -> Reshape/1
  Reshape/1 -> Out1/1

== system c10_wp_snake/controller/Subsystem17 ==
  In1 : Inport
  Demux1 : Demux  Outputs=3
  Mux5 : Mux  Inputs=2
  Reshape : Reshape  OutputDimensionality=Customize  OutputDimensions=[1,2]
  Terminator : Terminator
  Out1 : Outport
  wires:
  Reshape/1 -> Out1/1
  Mux5/1 -> Reshape/1
  Demux1/3 -> Terminator/1
  Demux1/2 -> Mux5/2
  Demux1/1 -> Mux5/1
  In1/1 -> Demux1/1

== system c10_wp_snake/controller/Subsystem18 ==
  In1 : Inport
  Demux1 : Demux  Outputs=3
  Mux5 : Mux  Inputs=2
  Reshape : Reshape  OutputDimensionality=Customize  OutputDimensions=[1,2]
  Terminator : Terminator
  Out1 : Outport
  wires:
  In1/1 -> Demux1/1
  Demux1/1 -> Mux5/1
  Demux1/2 -> Mux5/2
  Demux1/3 -> Terminator/1
  Mux5/1 -> Reshape/1
  Reshape/1 -> Out1/1

== system c10_wp_snake/controller/Subsystem2 ==
  note: Path Following with Obstacle Avoidance in Simulink
  Ranges : Inport
  Angels : Inport  Port=2
  Pose : Inport  Port=3
  WayPoints : Inport  Port=4
  Adjust Velocities to Avoid Obstacles : Subsystem
  Compute Velocity and Heading for Path following : Subsystem
  Constant1 : Constant  Value=scanAngles
  More Info : Subsystem
      settings: OpenFcn=showdemo(bdroot(gcb))
      mask Display: disp('?')
  Outputs : Subsystem
  v : Outport
  w : Outport  Port=2
  CloseToGoal : Outport  Port=3
  wires:
  Outputs/2(w) -> w/1
  Outputs/1(v) -> v/1
  Adjust Velocities to Avoid Obstacles/1(dV) -> Outputs/1(dV)
  Compute Velocity and Heading for Path following/4(CloseToGoal) -> CloseToGoal/1, Outputs/5(CloseToGoal)
  WayPoints/1 -> Compute Velocity and Heading for Path following/2(Waypoints)
  Ranges/1 -> Adjust Velocities to Avoid Obstacles/1(Ranges)
  Compute Velocity and Heading for Path following/2(V) -> Adjust Velocities to Avoid Obstacles/4(V), Outputs/3(V)
  Adjust Velocities to Avoid Obstacles/2(dW) -> Outputs/2(dW)
  Pose/1 -> Compute Velocity and Heading for Path following/1(CurrentPose)
  Compute Velocity and Heading for Path following/3(W) -> Adjust Velocities to Avoid Obstacles/5(W), Outputs/4(W)
  Compute Velocity and Heading for Path following/1(TargetDir) -> Adjust Velocities to Avoid Obstacles/3(TargetDir)
  Angels/1 -> Adjust Velocities to Avoid Obstacles/2(Angles)

== system c10_wp_snake/controller/Subsystem3 ==
  note: Path Following with Obstacle Avoidance in Simulink
  Ranges : Inport
  Angels : Inport  Port=2
  Pose : Inport  Port=3
  WayPoints : Inport  Port=4
  Adjust Velocities to Avoid Obstacles : Subsystem
  Compute Velocity and Heading for Path following : Subsystem
  Constant1 : Constant  Value=scanAngles
  More Info : Subsystem
      settings: OpenFcn=showdemo(bdroot(gcb))
      mask Display: disp('?')
  Outputs : Subsystem
  v : Outport
  w : Outport  Port=2
  CloseToGoal : Outport  Port=3
  wires:
  Angels/1 -> Adjust Velocities to Avoid Obstacles/2(Angles)
  Compute Velocity and Heading for Path following/1(TargetDir) -> Adjust Velocities to Avoid Obstacles/3(TargetDir)
  Compute Velocity and Heading for Path following/3(W) -> Outputs/4(W), Adjust Velocities to Avoid Obstacles/5(W)
  Pose/1 -> Compute Velocity and Heading for Path following/1(CurrentPose)
  Adjust Velocities to Avoid Obstacles/2(dW) -> Outputs/2(dW)
  Compute Velocity and Heading for Path following/2(V) -> Outputs/3(V), Adjust Velocities to Avoid Obstacles/4(V)
  Ranges/1 -> Adjust Velocities to Avoid Obstacles/1(Ranges)
  WayPoints/1 -> Compute Velocity and Heading for Path following/2(Waypoints)
  Compute Velocity and Heading for Path following/4(CloseToGoal) -> Outputs/5(CloseToGoal), CloseToGoal/1
  Adjust Velocities to Avoid Obstacles/1(dV) -> Outputs/1(dV)
  Outputs/1(v) -> v/1
  Outputs/2(w) -> w/1

== system c10_wp_snake/controller/Subsystem4 ==
  note: Path Following with Obstacle Avoidance in Simulink
  Ranges : Inport
  Angels : Inport  Port=2
  Pose : Inport  Port=3
  WayPoints : Inport  Port=4
  Adjust Velocities to Avoid Obstacles : Subsystem
  Compute Velocity and Heading for Path following : Subsystem
  Constant1 : Constant  Value=scanAngles
  More Info : Subsystem
      settings: OpenFcn=showdemo(bdroot(gcb))
      mask Display: disp('?')
  Outputs : Subsystem
  v : Outport
  w : Outport  Port=2
  CloseToGoal : Outport  Port=3
  wires:
  Outputs/2(w) -> w/1
  Outputs/1(v) -> v/1
  Adjust Velocities to Avoid Obstacles/1(dV) -> Outputs/1(dV)
  Compute Velocity and Heading for Path following/4(CloseToGoal) -> CloseToGoal/1, Outputs/5(CloseToGoal)
  WayPoints/1 -> Compute Velocity and Heading for Path following/2(Waypoints)
  Ranges/1 -> Adjust Velocities to Avoid Obstacles/1(Ranges)
  Compute Velocity and Heading for Path following/2(V) -> Adjust Velocities to Avoid Obstacles/4(V), Outputs/3(V)
  Adjust Velocities to Avoid Obstacles/2(dW) -> Outputs/2(dW)
  Pose/1 -> Compute Velocity and Heading for Path following/1(CurrentPose)
  Compute Velocity and Heading for Path following/3(W) -> Adjust Velocities to Avoid Obstacles/5(W), Outputs/4(W)
  Compute Velocity and Heading for Path following/1(TargetDir) -> Adjust Velocities to Avoid Obstacles/3(TargetDir)
  Angels/1 -> Adjust Velocities to Avoid Obstacles/2(Angles)

== system c10_wp_snake/controller/Subsystem5 ==
  note: Path Following with Obstacle Avoidance in Simulink
  Ranges : Inport
  Angels : Inport  Port=2
  Pose : Inport  Port=3
  WayPoints : Inport  Port=4
  Adjust Velocities to Avoid Obstacles : Subsystem
  Compute Velocity and Heading for Path following : Subsystem
  Constant1 : Constant  Value=scanAngles
  More Info : Subsystem
      settings: OpenFcn=showdemo(bdroot(gcb))
      mask Display: disp('?')
  Outputs : Subsystem
  v : Outport
  w : Outport  Port=2
  CloseToGoal : Outport  Port=3
  wires:
  Angels/1 -> Adjust Velocities to Avoid Obstacles/2(Angles)
  Compute Velocity and Heading for Path following/1(TargetDir) -> Adjust Velocities to Avoid Obstacles/3(TargetDir)
  Compute Velocity and Heading for Path following/3(W) -> Outputs/4(W), Adjust Velocities to Avoid Obstacles/5(W)
  Pose/1 -> Compute Velocity and Heading for Path following/1(CurrentPose)
  Adjust Velocities to Avoid Obstacles/2(dW) -> Outputs/2(dW)
  Compute Velocity and Heading for Path following/2(V) -> Outputs/3(V), Adjust Velocities to Avoid Obstacles/4(V)
  Ranges/1 -> Adjust Velocities to Avoid Obstacles/1(Ranges)
  WayPoints/1 -> Compute Velocity and Heading for Path following/2(Waypoints)
  Compute Velocity and Heading for Path following/4(CloseToGoal) -> Outputs/5(CloseToGoal), CloseToGoal/1
  Adjust Velocities to Avoid Obstacles/1(dV) -> Outputs/1(dV)
  Outputs/1(v) -> v/1
  Outputs/2(w) -> w/1

== system c10_wp_snake/controller/Subsystem6 ==
  note: Path Following with Obstacle Avoidance in Simulink
  Ranges : Inport
  Angels : Inport  Port=2
  Pose : Inport  Port=3
  WayPoints : Inport  Port=4
  Adjust Velocities to Avoid Obstacles : Subsystem
  Compute Velocity and Heading for Path following : Subsystem
  Constant1 : Constant  Value=scanAngles
  More Info : Subsystem
      settings: OpenFcn=showdemo(bdroot(gcb))
      mask Display: disp('?')
  Outputs : Subsystem
  v : Outport
  w : Outport  Port=2
  CloseToGoal : Outport  Port=3
  wires:
  Outputs/2(w) -> w/1
  Outputs/1(v) -> v/1
  Adjust Velocities to Avoid Obstacles/1(dV) -> Outputs/1(dV)
  Compute Velocity and Heading for Path following/4(CloseToGoal) -> CloseToGoal/1, Outputs/5(CloseToGoal)
  WayPoints/1 -> Compute Velocity and Heading for Path following/2(Waypoints)
  Ranges/1 -> Adjust Velocities to Avoid Obstacles/1(Ranges)
  Compute Velocity and Heading for Path following/2(V) -> Adjust Velocities to Avoid Obstacles/4(V), Outputs/3(V)
  Adjust Velocities to Avoid Obstacles/2(dW) -> Outputs/2(dW)
  Pose/1 -> Compute Velocity and Heading for Path following/1(CurrentPose)
  Compute Velocity and Heading for Path following/3(W) -> Adjust Velocities to Avoid Obstacles/5(W), Outputs/4(W)
  Compute Velocity and Heading for Path following/1(TargetDir) -> Adjust Velocities to Avoid Obstacles/3(TargetDir)
  Angels/1 -> Adjust Velocities to Avoid Obstacles/2(Angles)

== system c10_wp_snake/controller/Subsystem7 ==
  note: Path Following with Obstacle Avoidance in Simulink
  Ranges : Inport
  Angels : Inport  Port=2
  Pose : Inport  Port=3
  WayPoints : Inport  Port=4
  Adjust Velocities to Avoid Obstacles : Subsystem
  Compute Velocity and Heading for Path following : Subsystem
  Constant1 : Constant  Value=scanAngles
  More Info : Subsystem
      settings: OpenFcn=showdemo(bdroot(gcb))
      mask Display: disp('?')
  Outputs : Subsystem
  v : Outport
  w : Outport  Port=2
  CloseToGoal : Outport  Port=3
  wires:
  Angels/1 -> Adjust Velocities to Avoid Obstacles/2(Angles)
  Compute Velocity and Heading for Path following/1(TargetDir) -> Adjust Velocities to Avoid Obstacles/3(TargetDir)
  Compute Velocity and Heading for Path following/3(W) -> Outputs/4(W), Adjust Velocities to Avoid Obstacles/5(W)
  Pose/1 -> Compute Velocity and Heading for Path following/1(CurrentPose)
  Adjust Velocities to Avoid Obstacles/2(dW) -> Outputs/2(dW)
  Compute Velocity and Heading for Path following/2(V) -> Outputs/3(V), Adjust Velocities to Avoid Obstacles/4(V)
  Ranges/1 -> Adjust Velocities to Avoid Obstacles/1(Ranges)
  WayPoints/1 -> Compute Velocity and Heading for Path following/2(Waypoints)
  Compute Velocity and Heading for Path following/4(CloseToGoal) -> Outputs/5(CloseToGoal), CloseToGoal/1
  Adjust Velocities to Avoid Obstacles/1(dV) -> Outputs/1(dV)
  Outputs/1(v) -> v/1
  Outputs/2(w) -> w/1

== system c10_wp_snake/controller/Subsystem8 ==
  note: Path Following with Obstacle Avoidance in Simulink
  Ranges : Inport
  Angels : Inport  Port=2
  Pose : Inport  Port=3
  WayPoints : Inport  Port=4
  Adjust Velocities to Avoid Obstacles : Subsystem
  Compute Velocity and Heading for Path following : Subsystem
  Constant1 : Constant  Value=scanAngles
  More Info : Subsystem
      settings: OpenFcn=showdemo(bdroot(gcb))
      mask Display: disp('?')
  Outputs : Subsystem
  v : Outport
  w : Outport  Port=2
  CloseToGoal : Outport  Port=3
  wires:
  Outputs/2(w) -> w/1
  Outputs/1(v) -> v/1
  Adjust Velocities to Avoid Obstacles/1(dV) -> Outputs/1(dV)
  Compute Velocity and Heading for Path following/4(CloseToGoal) -> CloseToGoal/1, Outputs/5(CloseToGoal)
  WayPoints/1 -> Compute Velocity and Heading for Path following/2(Waypoints)
  Ranges/1 -> Adjust Velocities to Avoid Obstacles/1(Ranges)
  Compute Velocity and Heading for Path following/2(V) -> Adjust Velocities to Avoid Obstacles/4(V), Outputs/3(V)
  Adjust Velocities to Avoid Obstacles/2(dW) -> Outputs/2(dW)
  Pose/1 -> Compute Velocity and Heading for Path following/1(CurrentPose)
  Compute Velocity and Heading for Path following/3(W) -> Adjust Velocities to Avoid Obstacles/5(W), Outputs/4(W)
  Compute Velocity and Heading for Path following/1(TargetDir) -> Adjust Velocities to Avoid Obstacles/3(TargetDir)
  Angels/1 -> Adjust Velocities to Avoid Obstacles/2(Angles)

== system c10_wp_snake/controller/Subsystem9 ==
  note: Path Following with Obstacle Avoidance in Simulink
  Ranges : Inport
  Angels : Inport  Port=2
  Pose : Inport  Port=3
  WayPoints : Inport  Port=4
  Adjust Velocities to Avoid Obstacles : Subsystem
  Compute Velocity and Heading for Path following : Subsystem
  Constant1 : Constant  Value=scanAngles
  More Info : Subsystem
      settings: OpenFcn=showdemo(bdroot(gcb))
      mask Display: disp('?')
  Outputs : Subsystem
  v : Outport
  w : Outport  Port=2
  CloseToGoal : Outport  Port=3
  wires:
  Angels/1 -> Adjust Velocities to Avoid Obstacles/2(Angles)
  Compute Velocity and Heading for Path following/1(TargetDir) -> Adjust Velocities to Avoid Obstacles/3(TargetDir)
  Compute Velocity and Heading for Path following/3(W) -> Outputs/4(W), Adjust Velocities to Avoid Obstacles/5(W)
  Pose/1 -> Compute Velocity and Heading for Path following/1(CurrentPose)
  Adjust Velocities to Avoid Obstacles/2(dW) -> Outputs/2(dW)
  Compute Velocity and Heading for Path following/2(V) -> Outputs/3(V), Adjust Velocities to Avoid Obstacles/4(V)
  Ranges/1 -> Adjust Velocities to Avoid Obstacles/1(Ranges)
  WayPoints/1 -> Compute Velocity and Heading for Path following/2(Waypoints)
  Compute Velocity and Heading for Path following/4(CloseToGoal) -> Outputs/5(CloseToGoal), CloseToGoal/1
  Adjust Velocities to Avoid Obstacles/1(dV) -> Outputs/1(dV)
  Outputs/1(v) -> v/1
  Outputs/2(w) -> w/1

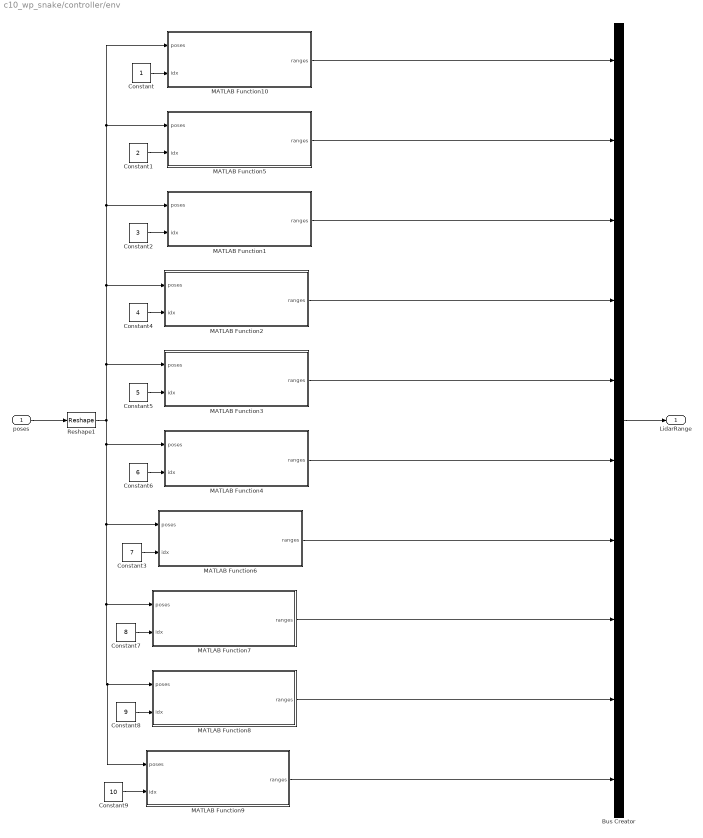
== system c10_wp_snake/controller/env ==
  poses : Inport
  Bus Creator : BusCreator  Inputs=10
  Constant : Constant
  Constant1 : Constant  Value=2
  Constant2 : Constant  Value=3
  Constant3 : Constant  Value=7
  Constant4 : Constant  Value=4
  Constant5 : Constant  Value=5
  Constant6 : Constant  Value=6
  Constant7 : Constant  Value=8
  Constant8 : Constant  Value=9
  Constant9 : Constant  Value=10
  MATLAB Function1 : MATLAB Function  TreatAsAtomicUnit=on
  MATLAB Function10 : MATLAB Function  TreatAsAtomicUnit=on
  MATLAB Function2 : MATLAB Function  TreatAsAtomicUnit=on
  MATLAB Function3 : MATLAB Function  TreatAsAtomicUnit=on
  MATLAB Function4 : MATLAB Function  TreatAsAtomicUnit=on
  MATLAB Function5 : MATLAB Function  TreatAsAtomicUnit=on
  MATLAB Function6 : MATLAB Function  TreatAsAtomicUnit=on
  MATLAB Function7 : MATLAB Function  TreatAsAtomicUnit=on
  MATLAB Function8 : MATLAB Function  TreatAsAtomicUnit=on
  MATLAB Function9 : MATLAB Function  TreatAsAtomicUnit=on
  Reshape1 : Reshape  OutputDimensionality=Customize  OutputDimensions=[3,10]
  LidarRange : Outport
  wires:
  MATLAB Function10/1(ranges) -> Bus Creator/1
  Bus Creator/1 -> LidarRange/1
  MATLAB Function5/1(ranges) -> Bus Creator/2
  MATLAB Function1/1(ranges) -> Bus Creator/3
  MATLAB Function2/1(ranges) -> Bus Creator/4
  MATLAB Function3/1(ranges) -> Bus Creator/5
  MATLAB Function4/1(ranges) -> Bus Creator/6
  MATLAB Function6/1(ranges) -> Bus Creator/7
  MATLAB Function7/1(ranges) -> Bus Creator/8
  MATLAB Function8/1(ranges) -> Bus Creator/9
  MATLAB Function9/1(ranges) -> Bus Creator/10
  Constant5/1 -> MATLAB Function3/2(idx)
  Constant/1 -> MATLAB Function10/2(idx)
  Constant6/1 -> MATLAB Function4/2(idx)
  Constant2/1 -> MATLAB Function1/2(idx)
  Constant1/1 -> MATLAB Function5/2(idx)
  poses/1 -> Reshape1/1
  Constant4/1 -> MATLAB Function2/2(idx)
  Constant3/1 -> MATLAB Function6/2(idx)
  Constant7/1 -> MATLAB Function7/2(idx)
  Reshape1/1 -> MATLAB Function3/1(poses), MATLAB Function2/1(poses), MATLAB Function1/1(poses), MATLAB Function5/1(poses), MATLAB Function10/1(poses), MATLAB Function4/1(poses), MATLAB Function6/1(poses), MATLAB Function7/1(poses), MATLAB Function9/1(poses), MATLAB Function8/1(poses)
  Constant8/1 -> MATLAB Function8/2(idx)
  Constant9/1 -> MATLAB Function9/2(idx)
